simulink model "SuspensionLinearFede"  (R2020a)
settings: Solver=VariableStepAuto  StartTime=0.0  StopTime=100  RelTol=1e-3
values from neighbouring files (symbols this model uses):
  A = eval(a)    [SuspensionFede.m]
  B = eval(b)    [SuspensionFede.m]
  K = lqr(A,B,Q,R)    [SuspensionFede.m]
  xe = transpose([z_ref vz_ref phi_ref wphi_ref theta_ref wtheta_ref ir1_ref ir2_ref ir3_ref ir4_ref ir5_ref ir6_ref qv_ref vqv_ref])    [SuspensionFede.m]
settings Model: Creator=Federico  LastModifiedBy=Federico

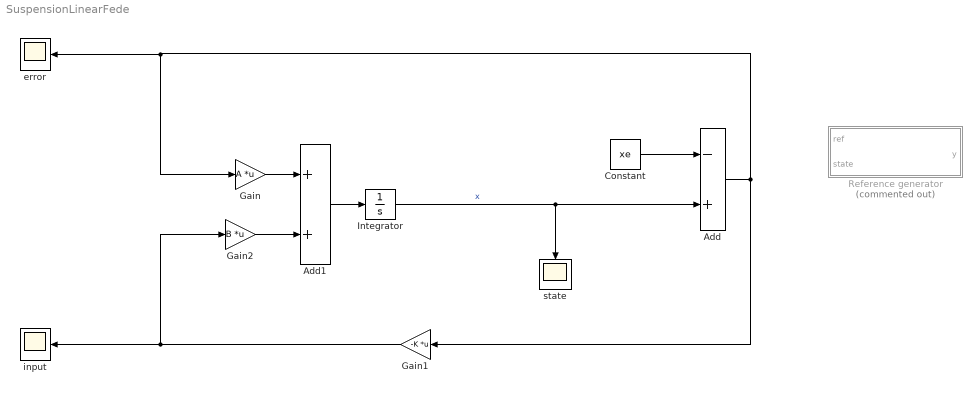
== system SuspensionLinearFede ==
  Add : Sum  Inputs=-+
  Add1 : Sum
  Constant : Constant  Value=xe
  Gain : Gain  Gain=A  Multiplication=Matrix(K*u)
  Gain1 : Gain  Gain=-K  Multiplication=Matrix(K*u)
  Gain2 : Gain  Gain=B  Multiplication=Matrix(K*u)
  Integrator : Integrator  ContinuousStateAttributes='iq1.id1.iq2.id2.v'
  Reference generator : MATLAB Function  Commented=on  TreatAsAtomicUnit=on
  error : Scope
  input : Scope
  state : Scope
  wires:
  Gain/1 -> Add1/1
  Add1/1 -> Integrator/1
  Gain1/1 -> Gain2/1, input/1
  Gain2/1 -> Add1/2
  Add/1 -> Gain/1, error/1, Gain1/1
  Integrator/1 -> Add/2, state/1  "x"
  Constant/1 -> Add/1

== matlab function SuspensionLinearFede/Reference generator ==
  data: y output; ref input; state input
function y = fcn(ref, state)

y = zeros(5,1);

%current references
y(1) = ref(1);
y(2) = ref(2);
y(3) = ref(3);
y(4) = ref(4);

y(5) = state(5);


v_ref = ref(5); % velocity v_reference
tollerance = 0.1; %needed to obtain a good final beaviour
accFactor = 0.1; %with this you can change the slope of the velocity and so the acceleration

%Speed ramp profile
if y(5) < v_ref - tollerance
    y(5)=(y(5)+accFactor);
elseif y(5) > v_ref + tollerance
    y(5)=(y(5)-accFactor);
else
    y(5)=v_ref;
end
